simulink model "sim"  (R2024b)
settings: Solver=VariableStepAuto  StartTime=0.0  StopTime=10.0  RelTol=1e-3
undefined symbols (not defined in the file or in its folder): b, k, M
settings Model: Creator=Ishak  LastModifiedBy=Ishak

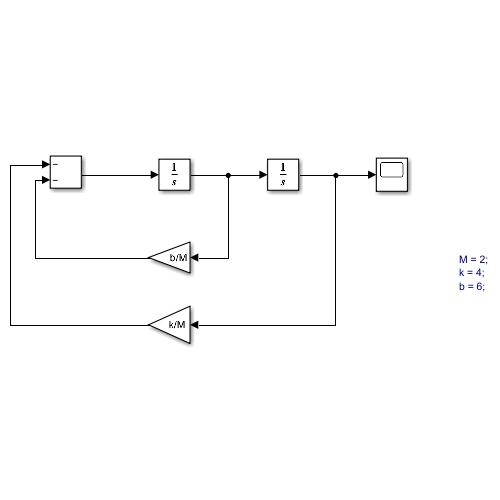
[thumbnail: Simulink's stored preview of the top-level diagram]
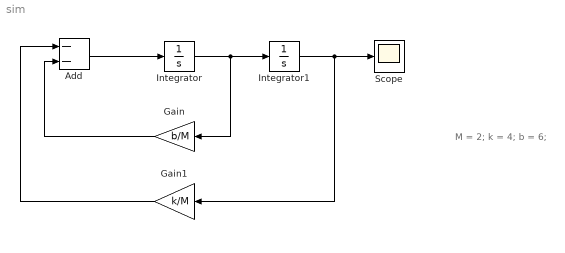
== system sim ==
  note: M = 2;
      | k = 4;
      | b = 6;
  Add : Sum  Inputs=--
  Gain : Gain  Gain=b/M
  Gain1 : Gain  Gain=k/M
  Integrator : Integrator
  Integrator1 : Integrator  InitialCondition=1
  Scope : Scope
  wires:
  Add/1 -> Integrator/1
  Integrator/1 -> Gain/1, Integrator1/1
  Integrator1/1 -> Gain1/1, Scope/1
  Gain/1 -> Add/2
  Gain1/1 -> Add/1
